simulink model "MPU9150_test"  (Simulink 9.2)
settings: Solver=FixedStepDiscrete  StartTime=0.0  StopTime=Inf  RelTol=1e-3  EnableMultiTasking=on
libraries: rpi_blkst x1
settings Model: Creator=jacques  LastModifiedBy=jacques  SimulationMode=external
settings OptimizationCC: ExpressionDepthLimit=2147483647  LifeSpan=1
settings DebuggingCC: SolverPrmCheckMsg=warning
settings HardwareCC: ProdLargestAtomicInteger=Long  ProdLargestAtomicFloat=Double  ProdIntDivRoundTo=Zero  ProdEndianess=LittleEndian  ProdHWDeviceType=ARM Compatible->ARM Cortex
settings SFSimCC: MATLABDynamicMemAlloc=off
settings RTWCC: SystemTargetFile=ert_rpi.tlc  TemplateMakefile=ert_rpi.tmf  PostCodeGenCommand=postGenFunc(buildInfo)  Description=RTW Embedded Coder RPI target
settings CodeAppCC: IgnoreCustomStorageClasses=off  CustomSymbolStrType=$N$R$M  InternalIdentifier=Classic
settings STFCustomTargetCC: ModelReferenceCompliant=off  CombineOutputUpdateFcns=on  ERTCustomFileBanners=on  SupportNonInlinedSFcns=off  RemoveResetFunc=on  MATLABClassNameForMDSCustomization=Simulink.SoftwareTarget.ERTCustomization  GRTInterface=off  SystemTargetFile=ert_rpi.tlc
settings ERTTargetCC: MultiwordLength=2048  ModelReferenceCompliant=off  ParMdlRefBuildCompliant=off  CompOptLevelCompliant=off  ConcurrentExecutionCompliant=off  SupportContinuousTime=on  ModelStepFunctionPrototypeControlCompliant=off  CPPClassGenCompliant=off  UseToolchainInfoCompliant=off  ExtMode=on  ExtModeMexArgs='192.168.2.1'  ERTCustomFileTemplate=ert_rpi_file_process.tlc  ConvertIfToSwitch=off  SuppressUnreachableDefaultCases=off

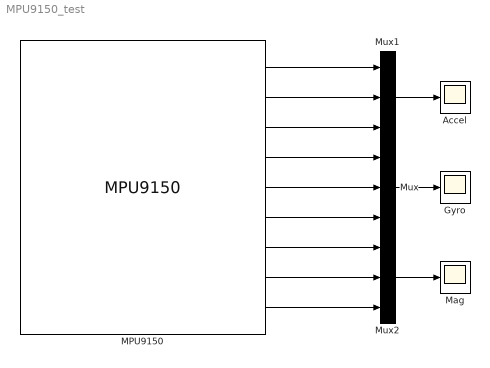
== system MPU9150_test ==
  Accel : Scope
  Gyro : Scope
  MPU9150 : rpi_blkst/MPU9150  rpi_mask_Ts=0.01
      settings: SourceProductName=RPI Blockset
  Mag : Scope
  Mux : Mux  Inputs=3
  Mux1 : Mux  Inputs=3
  Mux2 : Mux  Inputs=3
  wires:
  MPU9150/9 -> Mux2/3
  MPU9150/8 -> Mux2/2
  MPU9150/7 -> Mux2/1
  MPU9150/1 -> Mux1/1
  MPU9150/2 -> Mux1/2
  MPU9150/3 -> Mux1/3
  MPU9150/4 -> Mux/1
  MPU9150/5 -> Mux/2
  MPU9150/6 -> Mux/3
  Mux/1 -> Gyro/1
  Mux1/1 -> Accel/1
  Mux2/1 -> Mag/1
